simulink model "decoupled_simulation_pre"  (R2015b)
settings: Solver=ode45  StartTime=0.0  StopTime=10.0  RelTol=1e-3
values from neighbouring files (symbols this model uses):
  A = [0 1 0 0 ... (first row only)    [decoupled.m]
  B = [0 ; -0.286;0;0.386]    [decoupled.m]
  C = [1 0 0 0 ... (first row only)    [decoupled.m]
  D = [0 ; 0 ]    [decoupled.m]
  K = place(A,B,aim_poles)    [decoupled.m]
settings Model: Creator=16171  LastModifiedBy=fw-home
settings DataIOCC: LimitDataPoints=off
settings HardwareCC: ProdWordSize=32  ProdHWDeviceType=Specified
settings ModelReferenceCC: PropagateSignalLabelsOutOfModel=on
settings GRTTargetCC: GeneratePreprocessorConditionals=Disable all
settings ConfigComp: CovModelRefEnable=Off

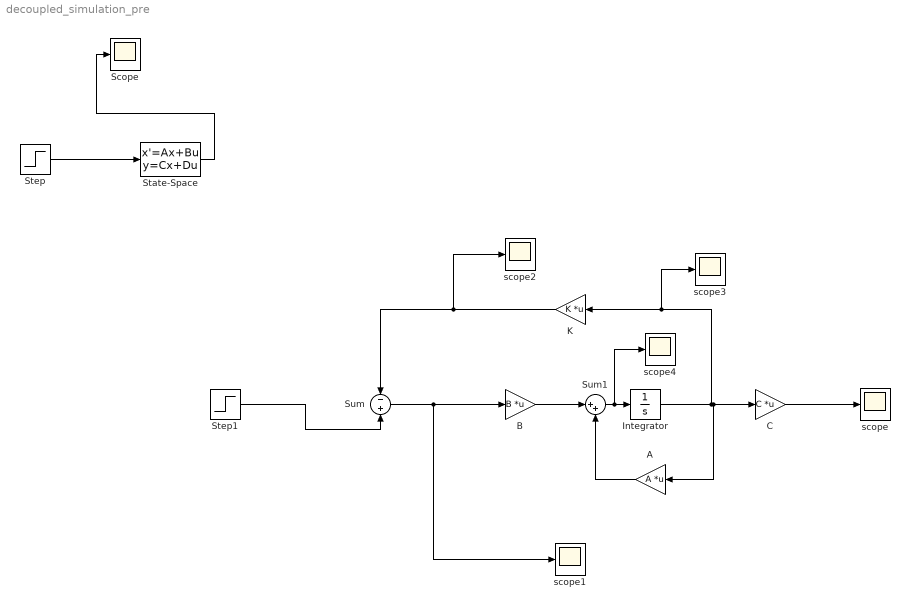
== system decoupled_simulation_pre ==
  A : Gain  Gain=A  Multiplication=Matrix(K*u)
  B : Gain  Gain=B  Multiplication=Matrix(K*u)
  C : Gain  Gain=C  Multiplication=Matrix(K*u)
  Integrator : Integrator
  K : Gain  Gain=K  Multiplication=Matrix(K*u)
  Scope : Scope
  State-Space : StateSpace  A=A  B=B  C=C  D=D  X0=[-0.1 0 0.1 0]
  Step : Step  After=0  SampleTime=0
  Step1 : Step  SampleTime=0
  Sum : Sum  Inputs=-+
  Sum1 : Sum  Inputs=|++
  scope{,1..4} (5 alike) : Scope
  wires:
  Step/1 -> State-Space/1
  State-Space/1 -> Scope/1
  Sum1/1 -> scope4/1, Integrator/1
  B/1 -> Sum1/1
  A/1 -> Sum1/2
  C/1 -> scope/1
  Integrator/1 -> scope3/1, K/1, A/1, C/1
  Step1/1 -> Sum/2
  K/1 -> scope2/1, Sum/1
  Sum/1 -> scope1/1, B/1
